simulink library "VSIGenLib"  (R2019b)
settings: Solver=VariableStepAuto  StartTime=0.0  StopTime=10.0  RelTol=1e-3
PostLoadFcn:
  | , if any(exist('dsrtsu_mdlpostloadfcn', 'file') ~= 0), dsrtsu_mdlpostloadfcn('Execute', bdroot); end,
undefined symbols (not defined in the file or in its folder): LIDAR, Ts_hil
libraries: simulink x76, $bdroot x46, etargetslib x30, ASCGenLib x26, dsmpblib x6
(part 1 of 3)
PreSaveFcn:
  | , if any(exist('dsmpb_private', 'file') ~= 0), dsmpb_private('dsmpb_mdlclblib', 'PreSave', bdroot); end,
CloseFcn:
  | , if any(exist('dsmpb_private', 'file') ~= 0), dsmpb_private('dsmpb_mdlclblib', 'Close', bdroot); end,
settings Model: DSRTSU_INTERNAL_RTI_VER=550  DSRTSU_INTERNAL_RTI_TYPE=rti1006  DSRTSU_INTERNAL_RTIFPGA=150  RTICANMMDATA=struct('GeneralSetupData',struct('modelroot',['C:\DEV_AREA\Dropbox (ORNL)\VSI_Projects\Bus_LDRD\Models\AutuBous\Libraries'],'generalsettings',struct('filesettings',struct('destfolder',struct('Name','RTICANMM_FILES','Check',1),'buildfolder',struct('Name','.','Check',1),'AbsDestfolder',struct('Name',['C:\DEV_AREA\Dropbox (ORNL)\VSI_Projects\Bus_LDRD\Models\AutuBous\Libraries\RTICANMM_FILES']),'AbsBuildfolder',struct('Name',['C:\DEV_AREA\Dropbox (ORNL)\VSI_Projects\Bus_LDRD\Models\AutuBous\Libraries']))),'options',struct('addpaths',1,'rmpaths',1,'addtrcexclusion',logical(1),'cannavigator',struct('checkmonitoring',0),'show_usrtrc',0,'use_usrtrc',0),'advanced',struct('options',[1 1 1 1 1 1 1 1 1 1 1 1 1 1 1 1 1 1 1 1 1 1 1 1 1 1 1 1 1 1 1 1 1 1 1 1 1 1 1 1 1 1 1 1 1 1 1 1 1 1 1 1 1 1 1 1 1 1 1 1 1 1 1 1 1 1 1 1 1 1 1 1 1 1 1 1 1 1 1 1 1 1 1 1 1 1 1 1 1 1 1 1 1 1 1 1 1 1 1 1]),'MPSetup',{{}},'modelname','ASCGenLib','block','ASCGenLib'))  DSMPB_ID_DATA={'3038',struct('BlockId','7554ba57-24ca-497c-8451-73d52e3b86d0','SignalIds',{{'d4c877d1-ebde-4f96-b2a8-0224649d3a55','7b23be26-dba1-46a4-8aa3-5f1a5d773025','7467d95a-e33c-43e0-80e0-b9ec821ea088','c4cc7553-c2bf-4d13-acf4-881d6e951a60','7e5f47f8-28e4-43cb-b5bf-dc1a0a661418'}}),'3039',struct('BlockId','2e587aad-7d58-4ac7-916d-d2cdf9db5fac','SignalIds',{{'4e86edab-e198-4349-a314-7708d2b89319','95d03380-f012-4c29-8404-e2860be7290e'}}),'3040',struct('BlockId','d0292f18-79e7-4173-b86f-1210574d231d','SignalIds',{{'8402872d-6d4c-4e14-a720-e068c4753129'}}),'3117',struct('BlockId','a65ad06e-9eda-4ae9-9547-95e074c45753','SignalIds',{{'82259da1-838b-488b-a89f-392b30c2e264','cfb0d8bc-2a97-4562-bcd4-a8450a074578','74b54aa3-9a67-4450-a3aa-2edc835e44ed','b9cfe27a-1c60-4148-bd3c-3991f4d00bba','739363a9-3c8a-4dd7-b6f2-72174523b9f2'}}),'3244',struct('BlockId','1c746f42-3a41-4f88-a84e-0b2f1d0a2ab7','SignalIds',{{'91fe521a-e6ea-4aaf-84fc-9c2a1af1ed6c','a7906f21-29de-4bc0-8fca-ca8bb9a7d91d'}}),'3245',struct('BlockId','ae8ced7c-16d4-43dd-b2cd-e42916ed1494','SignalIds',{{'4cc43c3b-8c61-403e-9c07-e3b753cfc380'}})}  Creator=ac0  LastModifiedBy=ac0
settings DataIOCC: ReturnWorkspaceOutputs=off
settings DebuggingCC: ArithmeticOperatorsInVariantConditions=warning
settings SFSimCC: SimUseLocalCustomCode=off  CustomCodeUndefinedFunction=UseInterfaceOnly
settings RTWCC: RTWUseLocalCustomCode=off
settings CodeAppCC: StateflowObjectComments=on

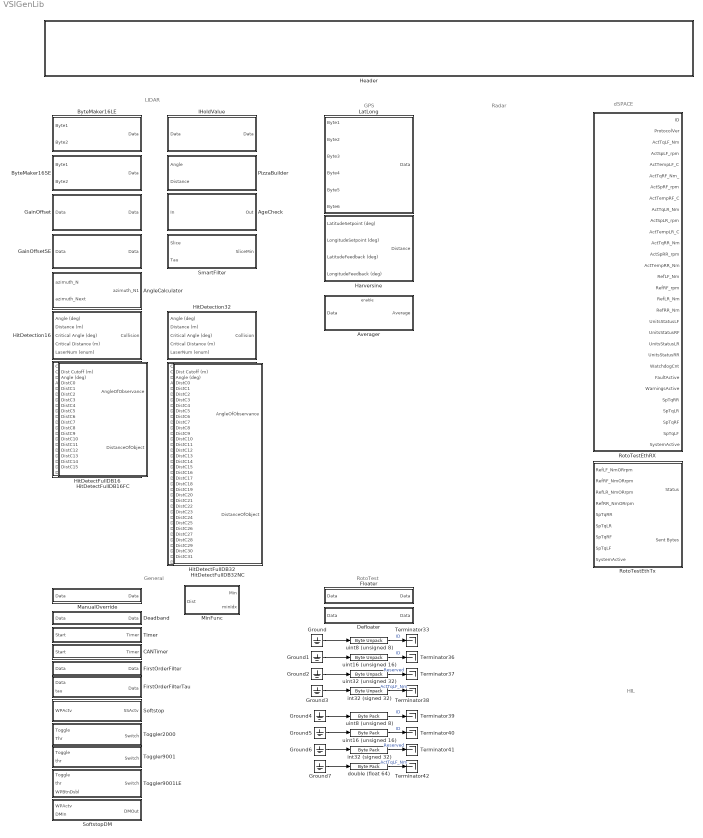
== system VSIGenLib ==
  note: LIDAR
  note: GPS
  note: Radar
  note: dSPACE
  note: General
  note: HIL
  note: RotoTest
  AgeCheck : Stateflow chart  TreatAsAtomicUnit=on
  AngleCalculator : MATLAB Function  TreatAsAtomicUnit=on
  Averager : Subsystem
      mask Display:
      | color('white')
      | disp('Averager')
      | port_label('input', 1, 'Data')
      | port_label('output', 1, 'Average')
      | % This block calculates an average only during enable. Block resets and
      | % recalculates when disabled and reenabled.
  ByteMaker16LE : Subsystem  mask{gain=1, offset=0}
      mask Display:
      | color('green')
      | disp('ByteMaker16LE')
      | port_label('input', 1, 'Byte1')
      | port_label('input', 2, 'Byte2')
      | port_label('output', 1, 'Data')
      | %This block takes to uint8 values and converts them to a uint16. Includes
      | %calibratable gain and offset.
  ByteMaker16SE : Subsystem  mask{gain=1, offset=0}
      mask Display:
      | color('green')
      | disp('ByteMaker16SE')
      | port_label('input', 1, 'Byte1')
      | port_label('input', 2, 'Byte2')
      | port_label('output', 1, 'Data')
      | %This block takes to uint8 values and converts them to a uint16, filtering
      | %for zeros. Includes calibratable gain and offset.
  CANTimer : Subsystem  mask{thr=0.05}
      mask prompts: thr "Threshold (s)"
      mask Display:
      | color('black')
      | disp('CAN Timer')
      | port_label('input', 1, 'Rx Time')
      | port_label('output', 1, 'CAN Ok')
      | %
  Deadband : Subsystem
      mask Display:
      | color('black')
      | disp('Deadband')
      | port_label('input', 1, 'Data')
      | port_label('output', 1, 'Data')
      | % Allows for a calibratable deadman across 0 for potentionmeters.
  Defloater : Subsystem
      mask Display:
      | color('black')
      | disp('Defloater')
      | port_label('input', 1, 'Data')
      | port_label('output', 1, 'Data')
      | % Converts a single floating point value to a vector of 4 uint8 values.
  FirstOrderFilter : Subsystem
      mask Display:
      | color('black')
      | disp('First Order Filter')
      | port_label('input', 1, 'Data')
      | port_label('output', 1, 'Data')
      | % First order filter
  FirstOrderFilterTau : Subsystem
      mask Display:
      | color('black')
      | disp('First Order Filter Tau')
      | port_label('input', 1, 'Data')
      | port_label('input', 2, 'Tau')
      | port_label('output', 1, 'Data')
      | % First order filter with calibratable tau
  Floater : Subsystem
      mask Display:
      | color('black')
      | disp('Floater')
      | port_label('input', 1, 'Data')
      | port_label('output', 1, 'Data')
      | % Converts a vector of 4 uint8 values to a single floating point value.
  GainOffset : Subsystem  mask{gain=1, offset=0}
      mask Display:
      | color('green')
      | disp('Gain/Offset')
      | port_label('input', 1, 'Data')
      | port_label('output', 1, 'Data')
  GainOffsetSE : Subsystem  mask{gain=0, offset=0}
      mask Display:
      | color('green')
      | disp('Gain/OffsetSE')
      | port_label('input', 1, 'Data')
      | port_label('output', 1, 'Data')
  Ground{,1..7} (8 alike) : Ground
  Harversine : Subsystem
      mask Display:
      | color('white')
      | disp('Harversine')
      | port_label('input', 1, 'y2 (deg)')
      | port_label('input', 2, 'x2 (deg)')
      | port_label('input', 3, 'y1 (deg)')
      | port_label('input', 4, 'x1 (deg)')
      | port_label('output', 1, 'Dist (ft)')
      | % This block calculates the great circle distance between two points.
  Header : Subsystem  mask{not='To act as a general library. Property of Adian Cook, Dean Deter and Oak Ridge National Laboratory.'}
      mask prompts: not "Notes"
      mask Display: disp([gcs '\n' not])
  HitDetectFullDB16 : Subsystem
      mask Display:
      | color('green')
      | disp('HitDetF16')
      | port_label('input', 1, 'Crit Az')
      | port_label('input', 2, 'Crit Dist (m)')
      | port_label('input', 3, 'Cutoff')
      | port_label('input', 4, 'Az')
      | port_label('input', 5, 'DistC0 (m)')
      | port_label('input', 6, 'DistC1 (m)')
      | port_label('input', 7, 'DistC2 (m)')
      | port_label('input', 8, 'DistC3 (m)')
      | port_label('input', 9, 'DistC4 (m)')
      | port_label('input', 10, 'DistC5 (m)')
      | port_label('input', 11, 'DistC6 (m)')
      | port_label('input', 12, 'DistC7 (m)')
      | port_label('input', 13, 'DistC8 (m)')
      | port_label('input', 14, 'DistC9 (m)')
      | port_label('input', 15, 'DistC10 (m)')
      | port_label('input', 16, 'DistC11 (m)')
      | port_label('input', 17, 'DistC12 (m)')
      | port_label('input', 18, 'DistC13 (m)')
      | port_label('input', 19, 'DistC14 (m)')
      | port_label('input', 20, 'DistC15 (m)')
      | port_label('output', 1, 'Hit (bool)')
      | port_label('output', 2, 'AOO (deg)')
      | port_label('output', 3, 'DOO (m)')
      | % More elegant version of 'Hit Detection' that does not need calibratable
      | % laser index. See mask parameters for 'Hit Detection' for help on this
      | % block.
  HitDetectFullDB16FC : Subsystem
      mask Display:
      | color('green')
      | disp('HitDetF16NC')
      | port_label('input', 1, 'Cutoff')
      | port_label('input', 2, 'Az')
      | port_label('input', 3, 'DistC0 (m)')
      | port_label('input', 4, 'DistC1 (m)')
      | port_label('input', 5, 'DistC2 (m)')
      | port_label('input', 6, 'DistC3 (m)')
      | port_label('input', 7, 'DistC4 (m)')
      | port_label('input', 8, 'DistC5 (m)')
      | port_label('input', 9, 'DistC6 (m)')
      | port_label('input', 10, 'DistC7 (m)')
      | port_label('input', 11, 'DistC8 (m)')
      | port_label('input', 12, 'DistC9 (m)')
      | port_label('input', 13, 'DistC10 (m)')
      | port_label('input', 14, 'DistC11 (m)')
      | port_label('input', 15, 'DistC12 (m)')
      | port_label('input', 16, 'DistC13 (m)')
      | port_label('input', 17, 'DistC14 (m)')
      | port_label('input', 18, 'DistC15 (m)')
      | port_label('output', 1, 'AOO (deg)')
      | port_label('output', 2, 'DOO (m)')
      | % More elegant version of 'Hit Detection' that does not need calibratable
      | % laser index. See mask parameters for 'Hit Detection' for help on this
      | % block. Does not have collision variables.
  HitDetectFullDB32 : Subsystem
      mask Display:
      | color('green')
      | disp('HitDetF32')
      | port_label('input', 1, 'Crit Az')
      | port_label('input', 2, 'Crit Dist (m)')
      | port_label('input', 3, 'Cutoff')
      | port_label('input', 4, 'Az')
      | port_label('input', 5, 'DistC0 (m)')
      | port_label('input', 6, 'DistC1 (m)')
      | port_label('input', 7, 'DistC2 (m)')
      | port_label('input', 8, 'DistC3 (m)')
      | port_label('input', 9, 'DistC4 (m)')
      | port_label('input', 10, 'DistC5 (m)')
      | port_label('input', 11, 'DistC6 (m)')
      | port_label('input', 12, 'DistC7 (m)')
      | port_label('input', 13, 'DistC8 (m)')
      | port_label('input', 14, 'DistC9 (m)')
      | port_label('input', 15, 'DistC10 (m)')
      | port_label('input', 16, 'DistC11 (m)')
      | port_label('input', 17, 'DistC12 (m)')
      | port_label('input', 18, 'DistC13 (m)')
      | port_label('input', 19, 'DistC14 (m)')
      | port_label('input', 20, 'DistC15 (m)')
      | port_label('input', 21, 'DistC0 (m)')
      | port_label('input', 22, 'DistC1 (m)')
      | port_label('input', 23, 'DistC2 (m)')
      | port_label('input', 24, 'DistC3 (m)')
      | port_label('input', 25, 'DistC4 (m)')
      | port_label('input', 26, 'DistC5 (m)')
      | port_label('input', 27, 'DistC6 (m)')
      | port_label('input', 28, 'DistC7 (m)')
      | port_label('input', 29, 'DistC8 (m)')
      | port_label('input', 30, 'DistC9 (m)')
      | port_label('input', 31, 'DistC10 (m)')
      | port_label('input', 32, 'DistC11 (m)')
      | port_label('input', 33, 'DistC12 (m)')
      | port_label('input', 34, 'DistC13 (m)')
      | port_label('input', 35, 'DistC14 (m)')
      | port_label('input', 36, 'DistC15 (m)')
      | port_label('output', 1, 'Hit (bool)')
      | port_label('output', 2, 'AOO (deg)')
      | port_label('output', 3, 'DOO (m)')
      | % More elegant version of 'Hit Detection' that does not need calibratable
      | % laser index. See mask parameters for 'Hit Detection' for help on this
      | % block.
  HitDetectFullDB32NC : Subsystem
      mask Display:
      | color('green')
      | disp('HitDetF32NC')
      | port_label('input', 1, 'Cutoff')
      | port_label('input', 2, 'Az')
      | port_label('input', 3, 'DistC0 (m)')
      | port_label('input', 4, 'DistC1 (m)')
      | port_label('input', 5, 'DistC2 (m)')
      | port_label('input', 6, 'DistC3 (m)')
      | port_label('input', 7, 'DistC4 (m)')
      | port_label('input', 8, 'DistC5 (m)')
      | port_label('input', 9, 'DistC6 (m)')
      | port_label('input', 10, 'DistC7 (m)')
      | port_label('input', 11, 'DistC8 (m)')
      | port_label('input', 12, 'DistC9 (m)')
      | port_label('input', 13, 'DistC10 (m)')
      | port_label('input', 14, 'DistC11 (m)')
      | port_label('input', 15, 'DistC12 (m)')
      | port_label('input', 16, 'DistC13 (m)')
      | port_label('input', 17, 'DistC14 (m)')
      | port_label('input', 18, 'DistC15 (m)')
      | port_label('input', 19, 'DistC0 (m)')
      | port_label('input', 20, 'DistC1 (m)')
      | port_label('input', 21, 'DistC2 (m)')
      | port_label('input', 22, 'DistC3 (m)')
      | port_label('input', 23, 'DistC4 (m)')
      | port_label('input', 24, 'DistC5 (m)')
      | port_label('input', 25, 'DistC6 (m)')
      | port_label('input', 26, 'DistC7 (m)')
      | port_label('input', 27, 'DistC8 (m)')
      | port_label('input', 28, 'DistC9 (m)')
      | port_label('input', 29, 'DistC10 (m)')
      | port_label('input', 30, 'DistC11 (m)')
      | port_label('input', 31, 'DistC12 (m)')
      | port_label('input', 32, 'DistC13 (m)')
      | port_label('input', 33, 'DistC14 (m)')
      | port_label('input', 34, 'DistC15 (m)')
      | port_label('output', 1, 'AOO (deg)')
      | port_label('output', 2, 'DOO (m)')
      | % More elegant version of 'Hit Detection' that does not need calibratable
      | % laser index. See mask parameters for 'Hit Detection' for help on this
      | % block. Does not have collision variables and allows handling downstream.
  HitDetection16 : Subsystem
      mask Display:
      | color('green')
      | disp('HitDetection16')
      | port_label('input', 1, 'Az')
      | port_label('input', 2, 'Dist (m)')
      | port_label('input', 3, 'Crit Az')
      | port_label('input', 4, 'Crit Dist (m)')
      | port_label('input', 5, 'LaserIdx (enum)')
      | port_label('output', 1, 'Hit (bool)')
      | % Used on single distance value with calibratable azimuth, distance, and
      | % laser ID. Block uses field of vision calibration and distance to detect a
      | % collision within field. For critcal azimuth, a calibration of 10 degrees
      | % would monitor between 350 and 10 (directly in front of LIDAR). Distance
      | % is calculated using a sine function to calculate 'r'.
  HitDetection32 : Subsystem
      mask Display:
      | color('green')
      | disp('HitDetection32')
      | port_label('input', 1, 'Az')
      | port_label('input', 2, 'Dist (m)')
      | port_label('input', 3, 'Crit Az')
      | port_label('input', 4, 'Crit Dist (m)')
      | port_label('input', 5, 'LaserIdx (enum)')
      | port_label('output', 1, 'Hit (bool)')
      | % Used on single distance value with calibratable azimuth, distance, and
      | % laser ID. Block uses field of vision calibration and distance to detect a
      | % collision within field. For critcal azimuth, a calibration of 10 degrees
      | % would monitor between 350 and 10 (directly in front of LIDAR). Distance
      | % is calculated using a sine function to calculate 'r'.
  IHoldValue : Subsystem
      mask Display:
      | color('green')
      | disp('HoldVal')
      | port_label('input', 1, 'Data')
      | port_label('output', 1, 'Data')
      | % Enables holding last non-zero value before value hits zero. Useful in LIDAR application
      | % as values consistently blip to zero.
  LatLong : Subsystem  mask{gain=1, offset=0}
      mask Display:
      | color('white')
      | disp('LatLong')
      | port_label('input', 1, 'Byte1')
      | port_label('input', 2, 'Byte2')
      | port_label('input', 3, 'Byte3')
      | port_label('input', 4, 'Byte4')
      | port_label('input', 5, 'Byte5')
      | port_label('input', 6, 'Byte6')
      | port_label('output', 1, 'Data')
      | % This block is used to decode the 48 bit message coming from the GPS.
      | % dSpace CAN Rx blocks cannot support messages greater than 4 bytes (32
      | % bits) so you must decode them manually. Block has ability to apply a
      | % manual gain and offset.
  ManualOverride : Subsystem
      mask Display:
      | color('black')
      | disp('Manual Override')
      | port_label('input', 1, 'Data')
      | port_label('output', 1, 'Data')
      | % Allows for manual override of any value in model.
  MinFunc : MATLAB Function  TreatAsAtomicUnit=on
  PizzaBuilder : Subsystem
      mask Display:
      | color('green')
      | disp('PizzaBuilder')
      | port_label('input', 1, 'Angle')
      | port_label('input', 2, 'Distance')
      | % Builds LIDAR slices.
  RotoTestEthRX : Subsystem
      mask Display:
      | color('white')
      | disp('RotTestEthTx')
      | port_label('output', 1, 'ID')
      | port_label('output', 2, 'ProtocolVer')
      | port_label('output', 3, 'ActTqLF (Nm)')
      | port_label('output', 4, 'RefRR_NmORrpm')
      | port_label('output', 5, 'ActTempLF (C)')
      | port_label('output', 6, 'ActTqRF (Nm)')
      | port_label('output', 7, 'ActSpRF (rpm)')
      | port_label('output', 8, 'ActTempRF (C)')
      | port_label('output', 9, 'ActTqLR (Nm)')
      | port_label('output', 10, 'ActSpLR (rpm)')
      | port_label('output', 11, 'ActTempLR (C)')
      | port_label('output', 12, 'ActTqRR (Nm)')
      | port_label('output', 13, 'ActSpRR (rpm)')
      | port_label('output', 14, 'ActTempRR (Nm)')
      | port_label('output', 15, 'RefLF (Nm)')
      | port_label('output', 16, 'RefRF (rpm)')
      | port_label('output', 17, 'RefLR (Nm)')
      | port_label('output', 18, 'RefRR (Nm)')
      | port_label('output', 19, 'UnitsStatusLF (enum)')
      | port_label('output', 20, 'UnitsStatusRF (enum)')
      | port_label('output', 21, 'UnitsStatusLR (enum)')
      | port_label('output', 22, 'UnitsStatusRR (enum)')
      | port_label('output', 23, 'WatchdogCnt (int)')
      | port_label('output', 24, 'FaultActive (enum)')
      | port_label('output', 25, 'WarningsActive (enum)')
      | port_label('output', 26, 'SpTqRR (enum)')
      | port_label('output', 27, 'SpTqLR (enum)')
      | port_label('output', 28, 'SpTqRF (enum)')
      | port_label('output', 29, 'SpTqLF (enum)')
      | port_label('output', 30, 'SystemActive (bool)')
  RotoTestEthTx : Subsystem
      mask Display:
      | color('white')
      | disp('RotTestEthTx')
      | port_label('input', 1, 'RefLF_NmORrpm')
      | port_label('input', 2, 'RefRF_NmORrpm')
      | port_label('input', 3, 'RefLR_NmORrpm')
      | port_label('input', 4, 'RefRR_NmORrpm')
      | port_label('input', 5, 'SqTrRR')
      | port_label('input', 6, 'SqTrLR')
      | port_label('input', 7, 'SqTrRF')
      | port_label('input', 8, 'SqTrLF')
      | port_label('input', 9, 'SystemActive')
      | port_label('output', 1, 'Status (bool)')
      | port_label('output', 2, 'Sent Bytes (int)')
  SmartFilter : Subsystem
      mask Display:
      | color('green')
      | disp('SmartFilter')
      | port_label('input', 1, 'Slice')
      | port_label('input', 2, 'Tau')
      | port_label('output', 1, 'SliceMin')
  Softstop : Stateflow chart  TreatAsAtomicUnit=on
  SoftstopDM : Stateflow chart  TreatAsAtomicUnit=on
  Terminator{33,36..42} (8 alike) : Terminator
  Timer : Subsystem
      mask Display:
      | color('black')
      | disp('Timer')
      | port_label('input', 1, 'Start')
      | port_label('output', 1, 'Timer')
      | %
  Toggler2000 : Stateflow chart  TreatAsAtomicUnit=on
  Toggler9001 : Stateflow chart  TreatAsAtomicUnit=on
  Toggler9001LE : Stateflow chart  TreatAsAtomicUnit=on
  "double (float 64) " : etargetslib/Byte Pack  datatypes={'double'}  byteAlign=1
      settings: SourceProductName=MATLAB Coder
  int32 (signed 32) : etargetslib/Byte Unpack  dimensions={[1]}  datatypes={'int32'}  byteAlign=1
      settings: SourceProductName=MATLAB Coder
  "int32 (signed 32) " : etargetslib/Byte Pack  datatypes={'int32'}  byteAlign=1
      settings: SourceProductName=MATLAB Coder
  uint16 (unsigned 16) : etargetslib/Byte Unpack  dimensions={[1]}  datatypes={'uint16'}  byteAlign=1
      settings: SourceProductName=MATLAB Coder
  "uint16 (unsigned 16) " : etargetslib/Byte Pack  datatypes={'uint16'}  byteAlign=1
      settings: SourceProductName=MATLAB Coder
  uint32 (unsigned 32) : etargetslib/Byte Unpack  dimensions={[1]}  datatypes={'uint32'}  byteAlign=1
      settings: SourceProductName=MATLAB Coder
  uint8 (unsigned 8) : etargetslib/Byte Unpack  dimensions={[1]}  datatypes={'uint8'}  byteAlign=1
      settings: SourceProductName=MATLAB Coder
  "uint8 (unsigned 8) " : etargetslib/Byte Pack  datatypes={'uint8'}  byteAlign=1
      settings: SourceProductName=MATLAB Coder
  wires:
  Ground3/1 -> int32 (signed 32)/1
  int32 (signed 32)/1 -> Terminator38/1  "ActTqLF_Nm"
  uint16 (unsigned 16)/1 -> Terminator36/1  "ID"
  Ground/1 -> uint8 (unsigned 8)/1
  Ground6/1 -> "int32 (signed 32) "/1
  "uint8 (unsigned 8) "/1 -> Terminator39/1  "ID"
  uint32 (unsigned 32)/1 -> Terminator37/1  "Reserved"
  Ground2/1 -> uint32 (unsigned 32)/1
  Ground5/1 -> "uint16 (unsigned 16) "/1
  Ground4/1 -> "uint8 (unsigned 8) "/1
  "double (float 64) "/1 -> Terminator42/1  "ActTqLF_Nm"
  "int32 (signed 32) "/1 -> Terminator41/1  "Reserved"
  Ground7/1 -> "double (float 64) "/1
  Ground1/1 -> uint16 (unsigned 16)/1
  "uint16 (unsigned 16) "/1 -> Terminator40/1  "ID"
  uint8 (unsigned 8)/1 -> Terminator33/1  "ID"

== system VSIGenLib/Averager ==
  Data : Inport
  Enable : EnablePort  StatesWhenEnabling=reset
  Constant : Constant
  Divide : Product  Inputs=*/
  Header : $bdroot/Header  not=''
  Sum : Sum  Inputs=|++
  Sum1 : Sum  Inputs=|++
  Unit Delay : UnitDelay  SampleTime=-1  HasFrameUpgradeWarning=on
  Unit Delay1 : UnitDelay  SampleTime=-1  HasFrameUpgradeWarning=on
  Average : Outport  VectorParamsAs1DForOutWhenUnconnected=off
  wires:
  Unit Delay/1 -> Sum/2
  Data/1 -> Sum/1
  Sum/1 -> Divide/1, Unit Delay/1
  Unit Delay1/1 -> Sum1/2
  Constant/1 -> Sum1/1
  Sum1/1 -> Unit Delay1/1, Divide/2
  Divide/1 -> Average/1

== system VSIGenLib/ByteMaker16LE ==
  Byte1 : Inport
  Byte2 : Inport  Port=2
  Add : Sum  Inputs=++++
  Constant : Constant  Value=offset
  Data Type Conversion : DataTypeConversion  OutDataTypeStr=uint8
  Data Type Conversion1 : DataTypeConversion  OutDataTypeStr=uint8
  Data Type Conversion2 : DataTypeConversion  OutDataTypeStr=single
  Extract Bits : simulink/Logic and Bit Operations/Extract Bits  bitsToExtract=Lower half  numBits=8  bitIdxRange=[0 7]  outScalingMode=Treat bit field as an integer
      settings: SourceProductName=Simulink
  Extract Bits1 : simulink/Logic and Bit Operations/Extract Bits  bitsToExtract=Upper half  numBits=8  bitIdxRange=[0 7]  outScalingMode=Treat bit field as an integer
      settings: SourceProductName=Simulink
  Extract Bits2 : simulink/Logic and Bit Operations/Extract Bits  bitsToExtract=Lower half  numBits=8  bitIdxRange=[0 7]  outScalingMode=Treat bit field as an integer
      settings: SourceProductName=Simulink
  Extract Bits3 : simulink/Logic and Bit Operations/Extract Bits  bitsToExtract=Upper half  numBits=8  bitIdxRange=[0 7]  outScalingMode=Treat bit field as an integer
      settings: SourceProductName=Simulink
  Gain : Gain  ParamDataTypeStr=uint16  OutDataTypeStr=uint16
  Gain1 : Gain  Gain=16  ParamDataTypeStr=uint16  OutDataTypeStr=uint16
  Gain2 : Gain  Gain=256  ParamDataTypeStr=uint16  OutDataTypeStr=uint16
  Gain3 : Gain  Gain=4096  ParamDataTypeStr=uint16  OutDataTypeStr=uint16
  Gain4 : Gain  Gain=gain  ParamDataTypeStr=double
  Header : $bdroot/Header  not=''
  Sum : Sum  Inputs=|++
  Data : Outport  VectorParamsAs1DForOutWhenUnconnected=off
  wires:
  Data Type Conversion/1 -> Extract Bits1/1, Extract Bits/1
  Data Type Conversion1/1 -> Extract Bits3/1, Extract Bits2/1
  Extract Bits1/1 -> Gain1/1
  Extract Bits/1 -> Gain/1
  Extract Bits3/1 -> Gain3/1
  Extract Bits2/1 -> Gain2/1
  Gain1/1 -> Add/1
  Gain/1 -> Add/2
  Gain3/1 -> Add/3
  Gain2/1 -> Add/4
  Add/1 -> Gain4/1
  Byte1/1 -> Data Type Conversion/1
  Byte2/1 -> Data Type Conversion1/1
  Gain4/1 -> Sum/1
  Sum/1 -> Data Type Conversion2/1
  Constant/1 -> Sum/2
  Data Type Conversion2/1 -> Data/1

== system VSIGenLib/ByteMaker16SE ==
  Byte1 : Inport
  Byte2 : Inport  Port=2
  Add : Sum  Inputs=++++
  Constant : Constant  Value=offset
  Data Type Conversion : DataTypeConversion  OutDataTypeStr=uint8
  Data Type Conversion1 : DataTypeConversion  OutDataTypeStr=uint8
  Data Type Conversion2 : DataTypeConversion  OutDataTypeStr=single
  Extract Bits : simulink/Logic and Bit Operations/Extract Bits  bitsToExtract=Lower half  numBits=8  bitIdxRange=[0 7]  outScalingMode=Treat bit field as an integer
      settings: SourceProductName=Simulink
  Extract Bits1 : simulink/Logic and Bit Operations/Extract Bits  bitsToExtract=Upper half  numBits=8  bitIdxRange=[0 7]  outScalingMode=Treat bit field as an integer
      settings: SourceProductName=Simulink
  Extract Bits2 : simulink/Logic and Bit Operations/Extract Bits  bitsToExtract=Lower half  numBits=8  bitIdxRange=[0 7]  outScalingMode=Treat bit field as an integer
      settings: SourceProductName=Simulink
  Extract Bits3 : simulink/Logic and Bit Operations/Extract Bits  bitsToExtract=Upper half  numBits=8  bitIdxRange=[0 7]  outScalingMode=Treat bit field as an integer
      settings: SourceProductName=Simulink
  Gain : Gain  ParamDataTypeStr=uint16  OutDataTypeStr=uint16
  Gain1 : Gain  Gain=16  ParamDataTypeStr=uint16  OutDataTypeStr=uint16
  Gain2 : Gain  Gain=256  ParamDataTypeStr=uint16  OutDataTypeStr=uint16
  Gain3 : Gain  Gain=4096  ParamDataTypeStr=uint16  OutDataTypeStr=uint16
  Gain4 : Gain  Gain=gain  ParamDataTypeStr=double
  Header : $bdroot/Header  not=''
  IHoldValue : ASCGenLib/IHoldValue  SystemSampleTime=-1
  Sum : Sum  Inputs=|++
  Data : Outport  VectorParamsAs1DForOutWhenUnconnected=off
  wires:
  Data Type Conversion/1 -> Extract Bits1/1, Extract Bits/1
  Data Type Conversion1/1 -> Extract Bits3/1, Extract Bits2/1
  Extract Bits1/1 -> Gain1/1
  Extract Bits/1 -> Gain/1
  Extract Bits3/1 -> Gain3/1
  Extract Bits2/1 -> Gain2/1
  Gain1/1 -> Add/1
  Gain/1 -> Add/2
  Gain3/1 -> Add/3
  Gain2/1 -> Add/4
  Add/1 -> Gain4/1
  Byte1/1 -> Data Type Conversion/1
  Byte2/1 -> Data Type Conversion1/1
  Gain4/1 -> Sum/1
  Sum/1 -> IHoldValue/1
  Constant/1 -> Sum/2
  IHoldValue/1 -> Data Type Conversion2/1
  Data Type Conversion2/1 -> Data/1

== system VSIGenLib/CANTimer ==
  Start : Inport
  Compare To Constant : simulink/Logic and Bit Operations/Compare To Constant  relop=<=  const=thr  OutDataTypeStr=boolean
  Header : $bdroot/Header  not=''
  Memory : Memory  InheritSampleTime=on
  Memory1 : Memory  InheritSampleTime=on
  Relational Operator : RelationalOperator  Operator===  OutDataTypeStr=boolean  RndMeth=Nearest
  Sum : Sum  Inputs=|++
  Switch : Switch  Criteria=u2 ~= 0
  Ts_hil : Constant  Value=Ts_hil
  Zero : Constant  Value=0
  Timer : Outport  VectorParamsAs1DForOutWhenUnconnected=off
  wires:
  Switch/1 -> Memory1/1
  Relational Operator/1 -> Switch/2
  Zero/1 -> Switch/3
  Memory1/1 -> Compare To Constant/1, Sum/2
  Sum/1 -> Switch/1
  Ts_hil/1 -> Sum/1
  Memory/1 -> Relational Operator/2
  Start/1 -> Memory/1, Relational Operator/1
  Compare To Constant/1 -> Timer/1

== system VSIGenLib/Deadband ==
  Data : Inport
  DeadbandCenter : Constant  Value=0
  DeadbandWidth : Constant  Value=0.1
  Header : $bdroot/Header  not=''
  Logical Operator : Logic  Operator=OR  AllPortsSameDT=off  OutDataTypeStr=boolean
  Multiport Switch : MultiPortSwitch  DataPortOrder=Zero-based contiguous  Inputs=2  zeroidx=on
  Relational Operator : RelationalOperator  Operator=>  OutDataTypeStr=boolean  RndMeth=Simplest
  Relational Operator1 : RelationalOperator  Operator=<  OutDataTypeStr=boolean  RndMeth=Simplest
  Sum : Sum  Inputs=|++
  Sum1 : Sum  Inputs=|-+
  "Data " : Outport  VectorParamsAs1DForOutWhenUnconnected=off
  wires:
  Data/1 -> Relational Operator1/1, Relational Operator/1, Multiport Switch/3
  Sum1/1 -> Relational Operator1/2
  Logical Operator/1 -> Multiport Switch/1
  DeadbandCenter/1 -> Sum1/2, Multiport Switch/2, Sum/2
  Sum/1 -> Relational Operator/2
  Relational Operator/1 -> Logical Operator/2
  Relational Operator1/1 -> Logical Operator/1
  Multiport Switch/1 -> "Data "/1
  DeadbandWidth/1 -> Sum/1, Sum1/1

== system VSIGenLib/Defloater ==
  Data : Inport
  Defloater : MATLAB Function  TreatAsAtomicUnit=on
  Header : $bdroot/Header  not='To act as a general library. Property of Adian Cook, Dean Deter and Oak Ridge National Laboratory.'
  Mux : Mux
  "Data " : Outport
  wires:
  Data/1 -> Defloater/1(defloatMe)
  Defloater/4(byte4) -> Mux/4
  Defloater/1(byte1) -> Mux/1
  Defloater/2(byte2) -> Mux/2
  Defloater/3(byte3) -> Mux/3
  Mux/1 -> "Data "/1

== system VSIGenLib/FirstOrderFilter ==
  Data : Inport
  Add : Sum
  Data Type Conversion : DataTypeConversion  OutDataTypeStr=single
  Divide1 : Product  Inputs=*/
  Header : $bdroot/Header  not=''
  Memory : Memory  InheritSampleTime=on
  MinMax : MinMax  Function=max  Inputs=2
  Product : Product  RndMeth=Zero
  Product2 : Product  RndMeth=Zero
  Sum3 : Sum  Inputs=|+-
  dt : Constant  Value=0.001
  one : Constant
  tau : Constant  Value=0.004
  "Data " : Outport  VectorParamsAs1DForOutWhenUnconnected=off
  wires:
  Divide1/1 -> Sum3/2, Product/2
  one/1 -> Sum3/1
  Sum3/1 -> Product2/1
  Product2/1 -> Add/2
  Add/1 -> Memory/1, Data Type Conversion/1
  Memory/1 -> Product2/2
  Product/1 -> Add/1
  Data/1 -> Product/1
  dt/1 -> Divide1/1, MinMax/1
  tau/1 -> MinMax/2
  MinMax/1 -> Divide1/2
  Data Type Conversion/1 -> "Data "/1

== system VSIGenLib/FirstOrderFilterTau ==
  Data : Inport
  tau : Inport  Port=2
  Add : Sum
  Data Type Conversion : DataTypeConversion  OutDataTypeStr=single
  Divide1 : Product  Inputs=*/
  Header : $bdroot/Header  not=''
  Memory : Memory  InheritSampleTime=on
  MinMax : MinMax  Function=max  Inputs=2
  Product : Product  RndMeth=Zero
  Product2 : Product  RndMeth=Zero
  Sum3 : Sum  Inputs=|+-
  dt : Constant  Value=0.001
  one : Constant
  "Data " : Outport  VectorParamsAs1DForOutWhenUnconnected=off
  wires:
  Divide1/1 -> Sum3/2, Product/2
  one/1 -> Sum3/1
  Sum3/1 -> Product2/1
  Product2/1 -> Add/2
  Add/1 -> Memory/1, Data Type Conversion/1
  Memory/1 -> Product2/2
  Product/1 -> Add/1
  Data/1 -> Product/1
  dt/1 -> Divide1/1, MinMax/1
  tau/1 -> MinMax/2
  MinMax/1 -> Divide1/2
  Data Type Conversion/1 -> "Data "/1

== system VSIGenLib/Floater ==
  Data : Inport
  Demux : Demux
  Floater : MATLAB Function  TreatAsAtomicUnit=on
  Header : $bdroot/Header  not='To act as a general library. Property of Adian Cook, Dean Deter and Oak Ridge National Laboratory.'
  "Data " : Outport
  wires:
  Floater/1(float32) -> "Data "/1
  Data/1 -> Demux/1
  Demux/4 -> Floater/4(byte4)
  Demux/3 -> Floater/3(byte3)
  Demux/2 -> Floater/2(byte2)
  Demux/1 -> Floater/1(byte1)

== system VSIGenLib/GainOffset ==
  Data : Inport
  Constant : Constant  Value=offset
  Gain4 : Gain  Gain=gain  ParamDataTypeStr=double
  Header : $bdroot/Header  not=''
  Sum : Sum  Inputs=|++
  "Data " : Outport  VectorParamsAs1DForOutWhenUnconnected=off
  wires:
  Data/1 -> Gain4/1
  Gain4/1 -> Sum/1
  Sum/1 -> "Data "/1
  Constant/1 -> Sum/2

== system VSIGenLib/GainOffsetSE ==
  Data : Inport
  Constant : Constant  Value=offset
  Gain4 : Gain  Gain=gain  ParamDataTypeStr=double
  Header : $bdroot/Header  not=''
  IHoldValue : $bdroot/IHoldValue  SystemSampleTime=-1  Latency=0  AutoFrameSizeCalculation=off
  Sum : Sum  Inputs=|++
  "Data " : Outport  VectorParamsAs1DForOutWhenUnconnected=off
  wires:
  Data/1 -> Gain4/1
  Gain4/1 -> Sum/1
  Sum/1 -> IHoldValue/1
  Constant/1 -> Sum/2
  IHoldValue/1 -> "Data "/1

== system VSIGenLib/Harversine ==
  note: https://www.movable-type.co.uk/scripts/latlong.html
  LatitudeSetpoint (deg) : Inport
  LongitudeSetpoint (deg) : Inport  Port=2
  LatitudeFeedback (deg) : Inport  Port=3
  LongitudeFeedback (deg) : Inport  Port=4
  2ft : Gain  Gain=6371e3*3.2808399  OutDataTypeStr=double
  Fcn1 : Fcn  Expr=2*atan2(sqrt(u(1)), sqrt(1-u(1)))
  Fcn5 : Fcn  Expr=sin(u(1)/2)*sin(u(1)/2)+cos(u(4))*cos(u(3))*sin(u(2)/2)*sin(u(2)/2)
  Header : $bdroot/Header  not=''
  Mux1 : Mux
  Subtract4 : Sum  Inputs=+-
  Subtract5 : Sum  Inputs=+-  AccumDataTypeStr=double  OutDataTypeStr=double
  deg2rad{,1..3} (4 alike) : Gain  Gain=pi/180  OutDataTypeStr=double
  Distance : Outport  VectorParamsAs1DForOutWhenUnconnected=off
  wires:
  deg2rad1/1 -> Subtract5/1  "LongitudeSetpoint"
  deg2rad/1 -> Subtract4/1, Mux1/3  "LatitudeSetpoint"
  deg2rad3/1 -> Subtract5/2  "LongitudeFeedback"
  Subtract4/1 -> Mux1/1  "dY Lat"
  Fcn5/1 -> Fcn1/1
  Mux1/1 -> Fcn5/1
  Fcn1/1 -> 2ft/1
  Subtract5/1 -> Mux1/2  "dX Long"
  deg2rad2/1 -> Subtract4/2, Mux1/4  "LatitudeFeedback"
  LatitudeSetpoint (deg)/1 -> deg2rad/1
  LatitudeFeedback (deg)/1 -> deg2rad2/1
  LongitudeSetpoint (deg)/1 -> deg2rad1/1
  LongitudeFeedback (deg)/1 -> deg2rad3/1
  2ft/1 -> Distance/1  "Distance (ft)"

== system VSIGenLib/Header ==

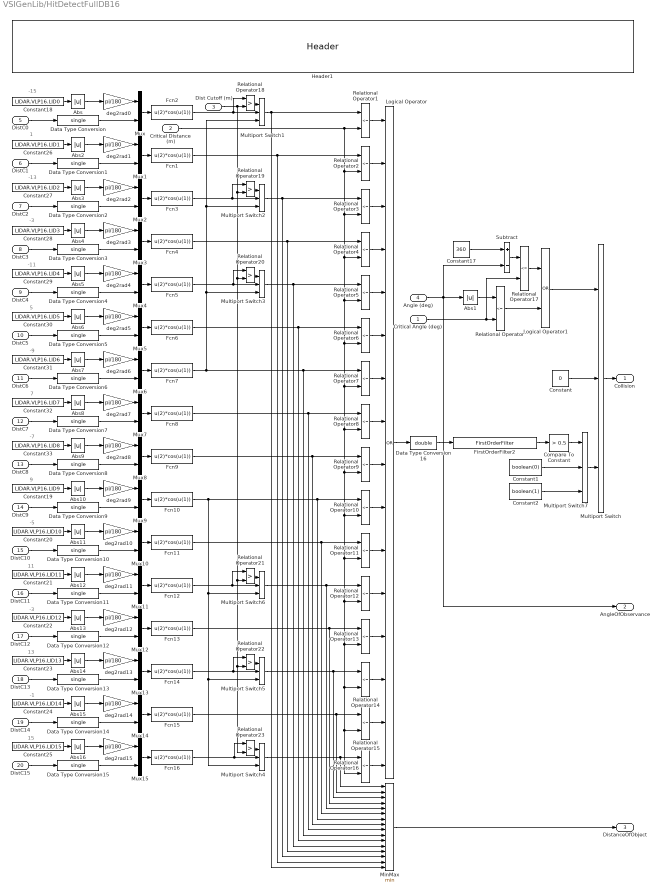
== system VSIGenLib/HitDetectFullDB16 ==
  note: -15
  note: 1
  note: -13
  note: -3
  note: -11
  note: 5
  note: -9
  note: 7
  note: -7
  note: 9
  note: -5
  note: 11
  note: 15
  note: -1
  note: 13
  note: -3
  Critical Angle (deg) : Inport
  Critical Distance (m) : Inport  Port=2
  Dist Cutoff (m) : Inport  Port=3
  Angle (deg) : Inport  Port=4
  DistC0 : Inport  Port=5
  DistC1 : Inport  Port=6
  DistC2 : Inport  Port=7
  DistC3 : Inport  Port=8
  DistC4 : Inport  Port=9
  DistC5 : Inport  Port=10
  DistC6 : Inport  Port=11
  DistC7 : Inport  Port=12
  DistC8 : Inport  Port=13
  DistC9 : Inport  Port=14
  DistC10 : Inport  Port=15
  DistC11 : Inport  Port=16
  DistC12 : Inport  Port=17
  DistC13 : Inport  Port=18
  DistC14 : Inport  Port=19
  DistC15 : Inport  Port=20
  Abs{,1..16} (17 alike) : Abs
  Compare To Constant : simulink/Logic and Bit Operations/Compare To Constant  relop=>  const=0.5  OutDataTypeStr=boolean
  Constant : Constant  Value=0
  Constant1 : Constant  Value=boolean(0)
  Constant17 : Constant  Value=360
  Constant18 : Constant  Value=LIDAR.VLP16.LID0
  Constant19 : Constant  Value=LIDAR.VLP16.LID9
  Constant2 : Constant  Value=boolean(1)
  Constant20 : Constant  Value=LIDAR.VLP16.LID10
  Constant21 : Constant  Value=LIDAR.VLP16.LID11
  Constant22 : Constant  Value=LIDAR.VLP16.LID12
  Constant23 : Constant  Value=LIDAR.VLP16.LID13
  Constant24 : Constant  Value=LIDAR.VLP16.LID14
  Constant25 : Constant  Value=LIDAR.VLP16.LID15
  Constant26 : Constant  Value=LIDAR.VLP16.LID1
  Constant27 : Constant  Value=LIDAR.VLP16.LID2
  Constant28 : Constant  Value=LIDAR.VLP16.LID3
  Constant29 : Constant  Value=LIDAR.VLP16.LID4
  Constant30 : Constant  Value=LIDAR.VLP16.LID5
  Constant31 : Constant  Value=LIDAR.VLP16.LID6
  Constant32 : Constant  Value=LIDAR.VLP16.LID7
  Constant33 : Constant  Value=LIDAR.VLP16.LID8
  Data Type Conversion{,1..15} (16 alike) : DataTypeConversion  OutDataTypeStr=single
  Data Type Conversion16 : DataTypeConversion  OutDataTypeStr=double
  Fcn{1..16} (16 alike) : Fcn  Expr=u(2)*cos(u(1))
  FirstOrderFilter2 : ASCGenLib/FirstOrderFilter  SystemSampleTime=-1
  Header1 : ASCGenLib/Header  not='L0 -15deg; L1 1deg; L2 -13deg; L3 -3deg; L4 -11deg; L5 5deg; L6 -9deg; L7 7deg; L8 -7deg; L9 9deg; L10 -5deg; L11 11deg; L12 -3deg; L13 13deg; L14 -1deg; L15 15deg'
  Logical Operator : Logic  Operator=OR  Inputs=16  AllPortsSameDT=off  OutDataTypeStr=boolean
  Logical Operator1 : Logic  Operator=OR  AllPortsSameDT=off  OutDataTypeStr=boolean
  MinMax : MinMax  Inputs=16
  Multiport Switch{,1..7} (8 alike) : MultiPortSwitch  DataPortOrder=Zero-based contiguous  Inputs=2  zeroidx=on
  Mux{,1..15} (16 alike) : Mux  Inputs=2
  Relational Operator{,1..17} (18 alike) : RelationalOperator  Operator=<=  OutDataTypeStr=boolean  RndMeth=Simplest
  Relational Operator{18..23} (6 alike) : RelationalOperator  Operator=>  OutDataTypeStr=boolean  RndMeth=Simplest
  Subtract : Sum  Inputs=+-
  deg2rad{0..15} (16 alike) : Gain  Gain=pi/180  OutDataTypeStr=single
  Collision : Outport  VectorParamsAs1DForOutWhenUnconnected=off
  AngleOfObservance : Outport  Port=2  VectorParamsAs1DForOutWhenUnconnected=off
  DistanceOfObject : Outport  Port=3  VectorParamsAs1DForOutWhenUnconnected=off
  wires:
  Angle (deg)/1 -> Abs1/1, Subtract/2, AngleOfObservance/1
  Critical Angle (deg)/1 -> Relational Operator17/2, Relational Operator/2
  Relational Operator/1 -> Logical Operator1/2
  Constant/1 -> Multiport Switch/2
  Multiport Switch/1 -> Collision/1
  Relational Operator1/1 -> Logical Operator/1
  Constant18/1 -> Abs/1
  Mux/1 -> Fcn2/1
  Abs/1 -> deg2rad0/1
  Multiport Switch1/1 -> MinMax/16, Relational Operator1/1
  Abs1/1 -> Relational Operator/1
  Constant26/1 -> Abs2/1
  Mux1/1 -> Fcn1/1
  Abs2/1 -> deg2rad1/1
  DistC0/1 -> Data Type Conversion/1
  DistC1/1 -> Data Type Conversion1/1
  Relational Operator2/1 -> Logical Operator/2
  Logical Operator/1 -> Data Type Conversion16/1
  Constant27/1 -> Abs3/1
  Mux2/1 -> Fcn3/1
  Abs3/1 -> deg2rad2/1
  Constant28/1 -> Abs4/1
  Mux3/1 -> Fcn4/1
  Abs4/1 -> deg2rad3/1
  Fcn4/1 -> MinMax/13, Relational Operator4/1
  DistC2/1 -> Data Type Conversion2/1
  DistC3/1 -> Data Type Conversion3/1
  Relational Operator3/1 -> Logical Operator/3
  Relational Operator4/1 -> Logical Operator/4
  Relational Operator5/1 -> Logical Operator/5
  Constant29/1 -> Abs5/1
  Abs5/1 -> deg2rad4/1
  Mux4/1 -> Fcn5/1
  deg2rad4/1 -> Mux4/1
  Multiport Switch3/1 -> MinMax/12, Relational Operator5/1
  Constant30/1 -> Abs6/1
  Abs6/1 -> deg2rad5/1
  Mux5/1 -> Fcn6/1
  deg2rad5/1 -> Mux5/1
  Fcn6/1 -> MinMax/11, Relational Operator6/1
  DistC4/1 -> Data Type Conversion4/1
  DistC5/1 -> Data Type Conversion5/1
  Relational Operator6/1 -> Logical Operator/6
  Constant31/1 -> Abs7/1
  Abs7/1 -> deg2rad6/1
  Mux6/1 -> Fcn7/1
  deg2rad6/1 -> Mux6/1
  Fcn7/1 -> Multiport Switch1/3, Multiport Switch2/3, Multiport Switch3/3, MinMax/10, Relational Operator7/1
  Constant32/1 -> Abs8/1
  Abs8/1 -> deg2rad7/1
  Mux7/1 -> Fcn8/1
  deg2rad7/1 -> Mux7/1
  Fcn8/1 -> MinMax/9, Relational Operator8/1
  DistC6/1 -> Data Type Conversion6/1
  DistC7/1 -> Data Type Conversion7/1
  Relational Operator7/1 -> Logical Operator/7
  Relational Operator8/1 -> Logical Operator/8
  Constant33/1 -> Abs9/1
  Abs9/1 -> deg2rad8/1
  Mux8/1 -> Fcn9/1
  deg2rad8/1 -> Mux8/1
  Fcn9/1 -> MinMax/8, Relational Operator9/1
  DistC8/1 -> Data Type Conversion8/1
  Relational Operator9/1 -> Logical Operator/9
  Relational Operator10/1 -> Logical Operator/10
  Constant19/1 -> Abs10/1
  Abs10/1 -> deg2rad9/1
  Mux9/1 -> Fcn10/1
  deg2rad9/1 -> Mux9/1
  Fcn10/1 -> Multiport Switch6/3, Multiport Switch5/3, Multiport Switch4/3, MinMax/7, Relational Operator10/1
  Constant20/1 -> Abs11/1
  Abs11/1 -> deg2rad10/1
  Mux10/1 -> Fcn11/1
  deg2rad10/1 -> Mux10/1
  Fcn11/1 -> MinMax/6, Relational Operator11/1
  DistC9/1 -> Data Type Conversion9/1
  DistC10/1 -> Data Type Conversion10/1
  Relational Operator11/1 -> Logical Operator/11
  Constant21/1 -> Abs12/1
  Abs12/1 -> deg2rad11/1
  Mux11/1 -> Fcn12/1
  deg2rad11/1 -> Mux11/1
  Multiport Switch6/1 -> MinMax/5, Relational Operator12/1
  Constant22/1 -> Abs13/1
  Abs13/1 -> deg2rad12/1
  Mux12/1 -> Fcn13/1
  deg2rad12/1 -> Mux12/1
  Fcn13/1 -> MinMax/4, Relational Operator13/1
  DistC11/1 -> Data Type Conversion11/1
  DistC12/1 -> Data Type Conversion12/1
  Relational Operator12/1 -> Logical Operator/12
  Relational Operator13/1 -> Logical Operator/13
  Constant23/1 -> Abs14/1
  Abs14/1 -> deg2rad13/1
  Mux13/1 -> Fcn14/1
  deg2rad13/1 -> Mux13/1
  Multiport Switch5/1 -> MinMax/3, Relational Operator14/1
  Constant24/1 -> Abs15/1
  Abs15/1 -> deg2rad14/1
  Mux14/1 -> Fcn15/1
  deg2rad14/1 -> Mux14/1
  Fcn15/1 -> MinMax/2, Relational Operator15/1
  DistC13/1 -> Data Type Conversion13/1
  DistC14/1 -> Data Type Conversion14/1
  Relational Operator14/1 -> Logical Operator/14
  Relational Operator15/1 -> Logical Operator/15
  Critical Distance (m)/1 -> Relational Operator2/2, Relational Operator6/2, Relational Operator7/2, Relational Operator8/2, Relational Operator9/2, Relational Operator10/2, Relational Operator11/2, Relational Operator12/2, Relational Operator13/2, Relational Operator14/2, Relational Operator15/2, Relational Operator16/2, Relational Operator5/2, Relational Operator4/2, Relational Operator3/2, Relational Operator1/2
  Constant25/1 -> Abs16/1
  Abs16/1 -> deg2rad15/1
  Mux15/1 -> Fcn16/1
  deg2rad15/1 -> Mux15/1
  Multiport Switch4/1 -> MinMax/1, Relational Operator16/1
  DistC15/1 -> Data Type Conversion15/1
  Relational Operator16/1 -> Logical Operator/16
  Constant17/1 -> Subtract/1
  Subtract/1 -> Relational Operator17/1
  Logical Operator1/1 -> Multiport Switch/1
  Relational Operator17/1 -> Logical Operator1/1
  deg2rad0/1 -> Mux/1
  deg2rad1/1 -> Mux1/1
  deg2rad2/1 -> Mux2/1
  deg2rad3/1 -> Mux3/1
  Data Type Conversion/1 -> Mux/2
  Data Type Conversion1/1 -> Mux1/2
  Data Type Conversion2/1 -> Mux2/2
  Data Type Conversion3/1 -> Mux3/2
  Data Type Conversion4/1 -> Mux4/2
  Data Type Conversion5/1 -> Mux5/2
  Data Type Conversion6/1 -> Mux6/2
  Data Type Conversion7/1 -> Mux7/2
  Data Type Conversion8/1 -> Mux8/2
  Data Type Conversion9/1 -> Mux9/2
  Data Type Conversion10/1 -> Mux10/2
  Data Type Conversion11/1 -> Mux11/2
  Data Type Conversion12/1 -> Mux12/2
  Data Type Conversion13/1 -> Mux13/2
  Data Type Conversion14/1 -> Mux14/2
  Data Type Conversion15/1 -> Mux15/2
  Fcn2/1 -> Relational Operator18/1, Multiport Switch1/2
  Relational Operator18/1 -> Multiport Switch1/1
  Multiport Switch2/1 -> MinMax/14, Relational Operator3/1
  Relational Operator19/1 -> Multiport Switch2/1
  Fcn3/1 -> Multiport Switch2/2, Relational Operator19/1
  Relational Operator20/1 -> Multiport Switch3/1
  Fcn5/1 -> Relational Operator20/1, Multiport Switch3/2
  Fcn16/1 -> Relational Operator23/1, Multiport Switch4/2
  Relational Operator23/1 -> Multiport Switch4/1
  Fcn1/1 -> MinMax/15, Relational Operator2/1
  Fcn14/1 -> Relational Operator22/1, Multiport Switch5/2
  Relational Operator22/1 -> Multiport Switch5/1
  Fcn12/1 -> Relational Operator21/1, Multiport Switch6/2
  Relational Operator21/1 -> Multiport Switch6/1
  Dist Cutoff (m)/1 -> Relational Operator23/2, Relational Operator22/2, Relational Operator21/2, Relational Operator20/2, Relational Operator19/2, Relational Operator18/2
  FirstOrderFilter2/1 -> Compare To Constant/1
  Multiport Switch7/1 -> Multiport Switch/3
  Constant1/1 -> Multiport Switch7/2
  Constant2/1 -> Multiport Switch7/3
  Data Type Conversion16/1 -> FirstOrderFilter2/1
  Compare To Constant/1 -> Multiport Switch7/1
  MinMax/1 -> DistanceOfObject/1

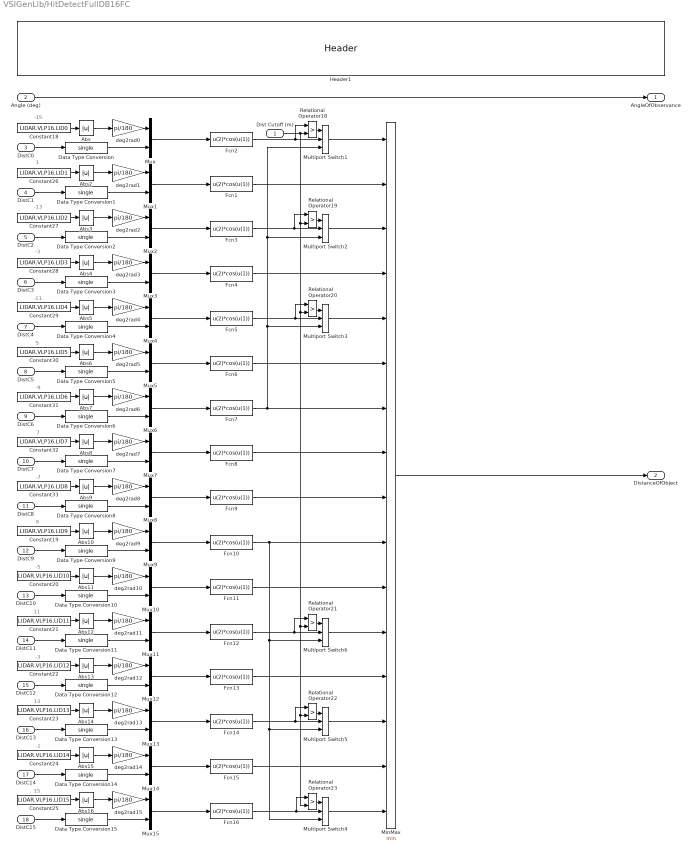
== system VSIGenLib/HitDetectFullDB16FC ==
  note: 1
  note: -1
  note: -9
  note: 11
  note: 9
  note: -5
  note: -11
  note: -7
  note: 7
  note: -15
  note: 13
  note: 15
  note: 5
  note: -3
  note: -3
  note: -13
  Dist Cutoff (m) : Inport
  Angle (deg) : Inport  Port=2
  DistC0 : Inport  Port=3
  DistC1 : Inport  Port=4
  DistC2 : Inport  Port=5
  DistC3 : Inport  Port=6
  DistC4 : Inport  Port=7
  DistC5 : Inport  Port=8
  DistC6 : Inport  Port=9
  DistC7 : Inport  Port=10
  DistC8 : Inport  Port=11
  DistC9 : Inport  Port=12
  DistC10 : Inport  Port=13
  DistC11 : Inport  Port=14
  DistC12 : Inport  Port=15
  DistC13 : Inport  Port=16
  DistC14 : Inport  Port=17
  DistC15 : Inport  Port=18
  Abs{,2..16} (16 alike) : Abs
  Constant18 : Constant  Value=LIDAR.VLP16.LID0
  Constant19 : Constant  Value=LIDAR.VLP16.LID9
  Constant20 : Constant  Value=LIDAR.VLP16.LID10
  Constant21 : Constant  Value=LIDAR.VLP16.LID11
  Constant22 : Constant  Value=LIDAR.VLP16.LID12
  Constant23 : Constant  Value=LIDAR.VLP16.LID13
  Constant24 : Constant  Value=LIDAR.VLP16.LID14
  Constant25 : Constant  Value=LIDAR.VLP16.LID15
  Constant26 : Constant  Value=LIDAR.VLP16.LID1
  Constant27 : Constant  Value=LIDAR.VLP16.LID2
  Constant28 : Constant  Value=LIDAR.VLP16.LID3
  Constant29 : Constant  Value=LIDAR.VLP16.LID4
  Constant30 : Constant  Value=LIDAR.VLP16.LID5
  Constant31 : Constant  Value=LIDAR.VLP16.LID6
  Constant32 : Constant  Value=LIDAR.VLP16.LID7
  Constant33 : Constant  Value=LIDAR.VLP16.LID8
  Data Type Conversion{,1..15} (16 alike) : DataTypeConversion  OutDataTypeStr=single
  Fcn{1..16} (16 alike) : Fcn  Expr=u(2)*cos(u(1))
  Header1 : ASCGenLib/Header  not='L0 -15deg; L1 1deg; L2 -13deg; L3 -3deg; L4 -11deg; L5 5deg; L6 -9deg; L7 7deg; L8 -7deg; L9 9deg; L10 -5deg; L11 11deg; L12 -3deg; L13 13deg; L14 -1deg; L15 15deg'
  MinMax : MinMax  Inputs=16
  Multiport Switch{1..6} (6 alike) : MultiPortSwitch  DataPortOrder=Zero-based contiguous  Inputs=2  zeroidx=on
  Mux{,1..15} (16 alike) : Mux  Inputs=2
  Relational Operator{18..23} (6 alike) : RelationalOperator  Operator=>  OutDataTypeStr=boolean  RndMeth=Simplest
  deg2rad{0..15} (16 alike) : Gain  Gain=pi/180  OutDataTypeStr=single
  AngleOfObservance : Outport  VectorParamsAs1DForOutWhenUnconnected=off
  DistanceOfObject : Outport  Port=2  VectorParamsAs1DForOutWhenUnconnected=off
  wires:
  Abs7/1 -> deg2rad6/1
  Abs10/1 -> deg2rad9/1
  Multiport Switch3/1 -> MinMax/5
  Mux2/1 -> Fcn3/1
  Mux4/1 -> Fcn5/1
  Relational Operator21/1 -> Multiport Switch6/1
  Data Type Conversion8/1 -> Mux8/2
  Multiport Switch2/1 -> MinMax/3
  Constant28/1 -> Abs4/1
  Fcn10/1 -> MinMax/10, Multiport Switch6/3, Multiport Switch5/3, Multiport Switch4/3
  Fcn9/1 -> MinMax/9
  Data Type Conversion4/1 -> Mux4/2
  Relational Operator19/1 -> Multiport Switch2/1
  Abs6/1 -> deg2rad5/1
  DistC9/1 -> Data Type Conversion9/1
  Constant33/1 -> Abs9/1
  Fcn8/1 -> MinMax/8
  Mux3/1 -> Fcn4/1
  Data Type Conversion13/1 -> Mux13/2
  Fcn12/1 -> Relational Operator21/1, Multiport Switch6/2
  deg2rad12/1 -> Mux12/1
  deg2rad9/1 -> Mux9/1
  DistC8/1 -> Data Type Conversion8/1
  Abs2/1 -> deg2rad1/1
  DistC15/1 -> Data Type Conversion15/1
  Data Type Conversion7/1 -> Mux7/2
  Constant24/1 -> Abs15/1
  Mux14/1 -> Fcn15/1
  Fcn6/1 -> MinMax/6
  deg2rad2/1 -> Mux2/1
  deg2rad13/1 -> Mux13/1
  Mux6/1 -> Fcn7/1
  Multiport Switch1/1 -> MinMax/1
  Data Type Conversion12/1 -> Mux12/2
  DistC5/1 -> Data Type Conversion5/1
  Fcn5/1 -> Relational Operator20/1, Multiport Switch3/2
  Abs15/1 -> deg2rad14/1
  Constant29/1 -> Abs5/1
  deg2rad5/1 -> Mux5/1
  Constant19/1 -> Abs10/1
  Fcn7/1 -> MinMax/7, Multiport Switch1/3, Multiport Switch2/3, Multiport Switch3/3
  Mux7/1 -> Fcn8/1
  DistC7/1 -> Data Type Conversion7/1
  Angle (deg)/1 -> AngleOfObservance/1
  Abs14/1 -> deg2rad13/1
  Mux9/1 -> Fcn10/1
  Multiport Switch5/1 -> MinMax/14
  Data Type Conversion14/1 -> Mux14/2
  Relational Operator18/1 -> Multiport Switch1/1
  DistC1/1 -> Data Type Conversion1/1
  MinMax/1 -> DistanceOfObject/1
  Abs5/1 -> deg2rad4/1
  Dist Cutoff (m)/1 -> Relational Operator23/2, Relational Operator22/2, Relational Operator21/2, Relational Operator20/2, Relational Operator19/2, Relational Operator18/2
  Constant23/1 -> Abs14/1
  deg2rad4/1 -> Mux4/1
  Relational Operator20/1 -> Multiport Switch3/1
  Data Type Conversion2/1 -> Mux2/2
  deg2rad6/1 -> Mux6/1
  Abs/1 -> deg2rad0/1
  Fcn1/1 -> MinMax/2
  DistC2/1 -> Data Type Conversion2/1
  deg2rad0/1 -> Mux/1
  Mux5/1 -> Fcn6/1
  Mux12/1 -> Fcn13/1
  Mux/1 -> Fcn2/1
  Constant21/1 -> Abs12/1
  DistC0/1 -> Data Type Conversion/1
  Mux10/1 -> Fcn11/1
  DistC4/1 -> Data Type Conversion4/1
  DistC13/1 -> Data Type Conversion13/1
  Fcn11/1 -> MinMax/11
  Relational Operator23/1 -> Multiport Switch4/1
  DistC11/1 -> Data Type Conversion11/1
  deg2rad14/1 -> Mux14/1
  Constant27/1 -> Abs3/1
  Abs8/1 -> deg2rad7/1
  deg2rad11/1 -> Mux11/1
  Data Type Conversion11/1 -> Mux11/2
  Mux11/1 -> Fcn12/1
  deg2rad8/1 -> Mux8/1
  Constant32/1 -> Abs8/1
  Abs3/1 -> deg2rad2/1
  Constant25/1 -> Abs16/1
  Constant20/1 -> Abs11/1
  DistC6/1 -> Data Type Conversion6/1
  Fcn15/1 -> MinMax/15
  Data Type Conversion6/1 -> Mux6/2
  DistC10/1 -> Data Type Conversion10/1
  Abs11/1 -> deg2rad10/1
  deg2rad3/1 -> Mux3/1
  Fcn4/1 -> MinMax/4
  Multiport Switch6/1 -> MinMax/12
  Fcn2/1 -> Relational Operator18/1, Multiport Switch1/2
  Abs4/1 -> deg2rad3/1
  Fcn14/1 -> Relational Operator22/1, Multiport Switch5/2
  Data Type Conversion10/1 -> Mux10/2
  Multiport Switch4/1 -> MinMax/16
  deg2rad15/1 -> Mux15/1
  Abs12/1 -> deg2rad11/1
  Data Type Conversion9/1 -> Mux9/2
  Mux1/1 -> Fcn1/1
  Mux15/1 -> Fcn16/1
  Fcn16/1 -> Relational Operator23/1, Multiport Switch4/2
  Fcn13/1 -> MinMax/13
  Constant26/1 -> Abs2/1
  DistC3/1 -> Data Type Conversion3/1
  Abs9/1 -> deg2rad8/1
  Constant31/1 -> Abs7/1
  deg2rad7/1 -> Mux7/1
  deg2rad1/1 -> Mux1/1
  Relational Operator22/1 -> Multiport Switch5/1
  DistC14/1 -> Data Type Conversion14/1
  Constant22/1 -> Abs13/1
  Data Type Conversion15/1 -> Mux15/2
  Constant30/1 -> Abs6/1
  Data Type Conversion1/1 -> Mux1/2
  Fcn3/1 -> Multiport Switch2/2, Relational Operator19/1
  Data Type Conversion/1 -> Mux/2
  Data Type Conversion3/1 -> Mux3/2
  DistC12/1 -> Data Type Conversion12/1
  Mux8/1 -> Fcn9/1
  Constant18/1 -> Abs/1
  Mux13/1 -> Fcn14/1
  Data Type Conversion5/1 -> Mux5/2
  Abs13/1 -> deg2rad12/1
  deg2rad10/1 -> Mux10/1
  Abs16/1 -> deg2rad15/1
